simulink model "ee_converter_ultracapacitor"  (R2020a)
settings: Solver=VariableStepAuto  StartTime=0.0  StopTime=15  MaxStep=0.1  RelTol=1e-3  EnableMultiTasking=on
PreLoadFcn:
  | Vref = 12;
StopFcn:
  | ee_addSimlogTimeStamp(bdroot)
libraries: fl_lib x12, nesl_utility x5, ee_lib x3
CloseFcn:
  | try,close(h1_ee_converter_ultracapacitor),end
  | clear h1_ee_converter_ultracapacitor
  | 
  | 
  | clear simlog_ee_converter_ultracapacitor
  | clear logsout_ee_converter_ultracapacitor
  | clear Vref tout
Description:
  | Ultracapacitor With Converter
settings Model: Creator=The MathWorks, Inc.  LastModifiedBy=sateeshk
settings DataIOCC: LimitDataPoints=on  MaxDataPoints=10000  SaveFormat=Array  ReturnWorkspaceOutputs=off  SignalLoggingName=logsout_ee_converter_ultracapacitor
settings OptimizationCC: ExpressionDepthLimit=2147483647  LifeSpan=inf
settings DebuggingCC: UnderspecifiedInitializationDetection=Classic  MergeDetectMultiDrivingBlocksExec=none  SolverPrmCheckMsg=warning  StateNameClashWarn=warning  SFUnexpectedBacktrackingDiag=warning  SFNoUnconditionalDefaultTransitionDiag=warning  SFExecutionAtInitializationDiag=none  ArithmeticOperatorsInVariantConditions=warning
settings HardwareCC: ProdBitPerPointer=32  ProdBitPerSizeT=32  ProdBitPerPtrDiffT=32  ProdLargestAtomicFloat=None  ProdIntDivRoundTo=Undefined  ProdEndianess=Unspecified  ProdWordSize=32  ProdHWDeviceType=32-bit Generic
settings ModelReferenceCC: PropagateSignalLabelsOutOfModel=off
settings SFSimCC: SimUseLocalCustomCode=off  CustomCodeUndefinedFunction=UseInterfaceOnly
settings RTWCC: RTWUseLocalCustomCode=off
settings CodeAppCC: StateflowObjectComments=on
settings GRTTargetCC: TargetLangStandard=C89/C90 (ANSI)
settings ConfigComp: CovMetricSettings=dw  CovHtmlReporting=on  CovSaveCumulativeToWorkspaceVar=on  CovSaveSingleToWorkspaceVar=on  CovExternalEMLEnable=off  CovSFcnEnable=off
settings SimscapeCC: SimscapeLogType=all  SimscapeLogSimulationStatistics=on  SimscapeLogName=simlog_ee_converter_ultracapacitor  SimscapeLogDataHistory=10000

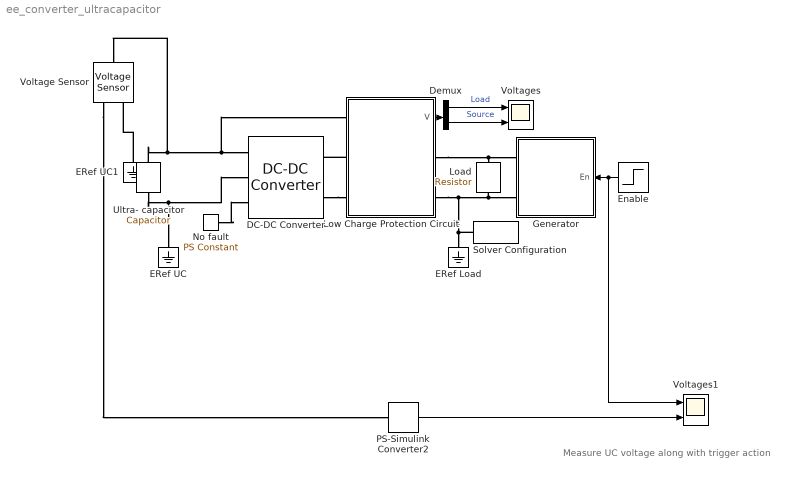
== system ee_converter_ultracapacitor ==
  note: Measure UC voltage along with trigger action
  DC-DC Converter : ee_lib/Semiconductors & Converters/Converters/DC-DC Converter  Vref_option=ee.enum.converters.voltageref.internal  v_ref=Vref V  P_rated=100 W  droop_param=1  droop=0.01 V/A  droop_percent=2  reversible=1  efficiency=95  P_fixed=0.1 W  model_dynamics=0  tau=0.02 s  v_ini=10 V  G_diode=1e-8 1/Ohm  i1_max=100 A  fault_condition=1  fault_threshold=0.5  thermal_mass=100 J/K  initial_temperature=298.15 K
      settings: SourceProductBaseCode=PS  InternalSimscapePortConfiguration="{\"Bottom\":[],\"Left\":[{\"id\":\"p1\",\"label\":\"1+\",\"type\":\"foundation.electrical.electrical\"},{\"id\":\"n1\",\"label\":\"1-\",\"type\":\"foundation.electrical.electrical\"},{\"id\":\"F\",\"label\":\"F\",\"type\":\"input\"}],\"Right\":[{\"id\":\"p2\",\"label\":\"2+\",\"type\":\"foundation.electrical.electrical\"},{\"id\":\"n2\",\"label\":\"2-\",\"type\":\"foundation.electrical.electrical\"}],\"Top\":[]}"
  Demux : Demux  Outputs=2
  ERef Load : fl_lib/Electrical/Electrical Elements/Electrical Reference
      settings: SourceProductBaseCode=MT,SS
  ERef UC : fl_lib/Electrical/Electrical Elements/Electrical Reference
      settings: SourceProductBaseCode=MT,SS
  ERef UC1 : fl_lib/Electrical/Electrical Elements/Electrical Reference
      settings: SourceProductBaseCode=MT,SS
  Enable : Step  Time=5  After=15  SampleTime=0
      settings: AttributesFormatString=On: %<Time> sec
  Generator : Subsystem
  Load : fl_lib/Electrical/Electrical Elements/Resistor  R=2 Ohm  i_specify=off  i_priority=High  i=0 A  i_nominal_specify=off  i_nominal_unit=A  i_nominal_value=1  v_specify=off  v_priority=High  v=0 V  v_nominal_specify=off  v_nominal_unit=V  v_nominal_value=1
      settings: SourceProductBaseCode=MT,SS
  Low Charge Protection Circuit : Subsystem  Tag=PublishSubsystem
  No fault : fl_lib/Physical Signals/Sources/PS Constant  constant=0
      settings: SourceProductBaseCode=MT,SS
  PS-Simulink Converter2 : nesl_utility/PS-Simulink Converter  PhysicalDomain=network_engine_domain  SubClassName=ps_output  LeftPortType=input  RightPortType=output  PseudoPeriodic=off  Frequencies=[]  Unit=1  AffineConversion=off
      settings: SourceProductBaseCode=MT,SS
  Solver Configuration : nesl_utility/Solver Configuration  PhysicalDomain=network_engine_domain  SubClassName=solver  LeftPortType=input  RightPortType=generic  Tones=[]  Harmonics=[]  SimulateNoise=off  Profile=off  UseLocalSampling=off  EnableSwitchedLinearOptims=on  FrequencyDomain=off  UseCCode=off  RelTol=0.001  AbsTol=1e-06  MinStep=1e-09  ToWorkspace=off  RevertToSquareIcSolve=off  NumHomotopyIterations=100  PhasorMode=off  PhasorModeNumHarmonics=1  DoDC=off  ResidualTolerance=1e-9  UseLocalSolver=off  LocalSolverChoice=NE_BACKWARD_EULER_ADVANCER  LocalSolverSampleTime=0.01  DoFixedCost=off  MaxNonlinIter=3  MaxModeIter=2  LinearAlgebra=auto  EquationFormulation=NE_TIME_EF  DelaysMemoryBudget=1024  AutomaticFiltering=on  FilteringTimeConstant=0.001  PartitionStorageMethod=AS_NEEDED  PartitionMemoryBudget=1024  PartitionMethod=FAST
      settings: SourceProductBaseCode=MT,SS
  Ultra- capacitor : fl_lib/Electrical/Electrical Elements/Capacitor  c=10 F  r=0 Ohm  g=0 1/Ohm  i_specify=off  i_priority=High  i=0 A  i_nominal_specify=off  i_nominal_unit=A  i_nominal_value=1  v_specify=off  v_priority=High  v=0 V  v_nominal_specify=off  v_nominal_unit=V  v_nominal_value=1  vc_specify=on  vc_priority=High  vc=10 V  vc_nominal_specify=off  vc_nominal_unit=V  vc_nominal_value=1
      settings: SourceProductBaseCode=MT,SS
  Voltage Sensor : fl_lib/Electrical/Electrical Sensors/Voltage Sensor
  Voltages : Scope  NumInputPorts=2
  Voltages1 : Scope  NumInputPorts=2
  wires:
  Enable/1 -> Voltages1/1, Generator/1(En)
  Low Charge Protection Circuit/1(V) -> Demux/1
  Demux/1 -> Voltages/1  "Load"
  Demux/2 -> Voltages/2  "Source"
  PS-Simulink Converter2/1 -> Voltages1/2
  connections:
  Ultra- capacitor/RConn1 -- DC-DC Converter/LConn2 -- ERef UC/LConn1
  Ultra- capacitor/LConn1 -- Low Charge Protection Circuit/LConn1 -- DC-DC Converter/LConn1 -- Voltage Sensor/LConn1
  Low Charge Protection Circuit/LConn2 -- DC-DC Converter/RConn1
  Low Charge Protection Circuit/RConn2 -- Solver Configuration/RConn1 -- ERef Load/LConn1 -- Generator/RConn2 -- Load/RConn1
  DC-DC Converter/RConn2 -- Low Charge Protection Circuit/LConn3
  Low Charge Protection Circuit/RConn1 -- Load/LConn1 -- Generator/RConn1
  No fault/RConn1 -- DC-DC Converter/LConn3
  ERef UC1/LConn1 -- Voltage Sensor/RConn2
  Voltage Sensor/RConn1 -- PS-Simulink Converter2/LConn1

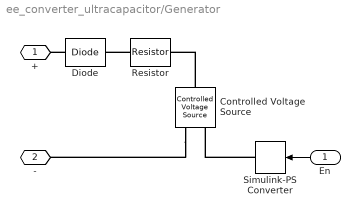
== system ee_converter_ultracapacitor/Generator ==
  En : Inport
  Controlled Voltage Source : fl_lib/Electrical/Electrical Sources/Controlled Voltage Source
      settings: SourceProductBaseCode=MT,SS
  Diode : fl_lib/Electrical/Electrical Elements/Diode  Vf=0.6 V  Ron=0.01 Ohm  Goff=1e-8 1/Ohm  i_specify=off  i_priority=High  i=0 A  i_nominal_specify=off  i_nominal_unit=A  i_nominal_value=1  v_specify=off  v_priority=High  v=0 V  v_nominal_specify=off  v_nominal_unit=V  v_nominal_value=1
      settings: SourceProductBaseCode=MT,SS
  Resistor : fl_lib/Electrical/Electrical Elements/Resistor  R=0.1 Ohm  i_specify=off  i_priority=High  i=0 A  i_nominal_specify=off  i_nominal_unit=A  i_nominal_value=1  v_specify=off  v_priority=High  v=0 V  v_nominal_specify=off  v_nominal_unit=V  v_nominal_value=1
      settings: SourceProductBaseCode=MT,SS
  Simulink-PS Converter : nesl_utility/Simulink-PS Converter  PhysicalDomain=network_engine_domain  SubClassName=ps_input  LeftPortType=input  RightPortType=output  PseudoPeriodic=off  Frequencies=[]  NoiseDistribution=none  NoiseParameters=[]  Unit=1  AffineConversion=off  FilteringAndDerivatives=zero  SimscapeFilterOrder=1  InputFilterTimeConstant=.001  UdotUserProvided=[]
      settings: SourceProductBaseCode=MT,SS
  + : PMIOPort  Side=Right
  - : PMIOPort  Port=2  Side=Right
  wires:
  En/1 -> Simulink-PS Converter/1
  connections:
  Controlled Voltage Source/RConn2 -- -/RConn1
  Simulink-PS Converter/RConn1 -- Controlled Voltage Source/RConn1
  Controlled Voltage Source/LConn1 -- Resistor/LConn1
  Diode/RConn1 -- +/RConn1
  Resistor/RConn1 -- Diode/LConn1

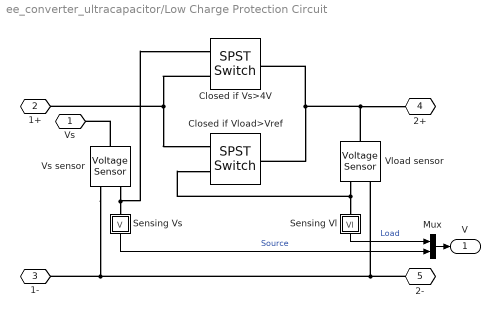
== system ee_converter_ultracapacitor/Low Charge Protection Circuit ==
  Closed if Vload>Vref : ee_lib/Switches & Breakers/SPST Switch  R_closed=0.01 Ohm  G_open=1e-6 S  Threshold=Vref V  Width=0.1 V  model_dynamics=0  t_on=0.001 s  t_off=0.001 s  initial_vT=0 V
      settings: SourceProductBaseCode=PS  InternalSimscapePortConfiguration="{\"Bottom\":[],\"Left\":[{\"id\":\"vT\",\"label\":\"vT\",\"type\":\"input\"},{\"id\":\"p\",\"label\":\"\",\"type\":\"foundation.electrical.electrical\"}],\"Right\":[{\"id\":\"n\",\"label\":\"\",\"type\":\"foundation.electrical.electrical\"}],\"Top\":[]}"
  Closed if Vs>4V : ee_lib/Switches & Breakers/SPST Switch  R_closed=0.01 Ohm  G_open=1e-6 S  Threshold=4 V  Width=0.1 V  model_dynamics=0  t_on=0.001 s  t_off=0.001 s  initial_vT=0 V
      settings: SourceProductBaseCode=PS  InternalSimscapePortConfiguration="{\"Bottom\":[],\"Left\":[{\"id\":\"vT\",\"label\":\"vT\",\"type\":\"input\"},{\"id\":\"p\",\"label\":\"\",\"type\":\"foundation.electrical.electrical\"}],\"Right\":[{\"id\":\"n\",\"label\":\"\",\"type\":\"foundation.electrical.electrical\"}],\"Top\":[]}"
  Mux : Mux  Inputs=2
  Sensing Vl : Subsystem
      mask Display: disp('Vl')
  Sensing Vs : Subsystem
      mask Display: disp('Vs')
  Vload sensor : fl_lib/Electrical/Electrical Sensors/Voltage Sensor
      settings: SourceProductBaseCode=MT,SS
  Vs sensor : fl_lib/Electrical/Electrical Sensors/Voltage Sensor
      settings: SourceProductBaseCode=MT,SS
  Vs : PMIOPort  Side=Left
  1+ : PMIOPort  Port=2  Side=Left
  1- : PMIOPort  Port=3  Side=Left
  2+ : PMIOPort  Port=4  Side=Right
  2- : PMIOPort  Port=5  Side=Right
  V : Outport  VectorParamsAs1DForOutWhenUnconnected=off
  wires:
  Sensing Vl/1(Vl) -> Mux/1  "Load"
  Mux/1 -> V/1
  Sensing Vs/1(V) -> Mux/2  "Source"
  connections:
  Vload sensor/LConn1 -- 2+/RConn1 -- Closed if Vload>Vref/RConn1 -- Closed if Vs>4V/RConn1
  2-/RConn1 -- Vload sensor/RConn2 -- Vs sensor/RConn2 -- 1-/RConn1
  Closed if Vs>4V/LConn2 -- Closed if Vload>Vref/LConn2 -- 1+/RConn1
  Vs sensor/LConn1 -- Vs/RConn1
  Vs sensor/RConn1 -- Closed if Vs>4V/LConn1 -- Sensing Vs/LConn1
  Vload sensor/RConn1 -- Closed if Vload>Vref/LConn1 -- Sensing Vl/LConn1

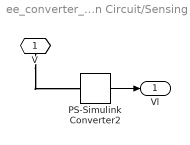
== system ee_converter_ultracapacitor/Low Charge Protection Circuit/Sensing Vl ==
  PS-Simulink Converter2 : nesl_utility/PS-Simulink Converter  PhysicalDomain=network_engine_domain  SubClassName=ps_output  LeftPortType=input  RightPortType=output  PseudoPeriodic=off  Frequencies=[]  Unit=1  AffineConversion=off
      settings: SourceProductBaseCode=MT,SS
  V : PMIOPort  Side=Left
  Vl : Outport  VectorParamsAs1DForOutWhenUnconnected=off
  wires:
  PS-Simulink Converter2/1 -> Vl/1
  connections:
  V/RConn1 -- PS-Simulink Converter2/LConn1

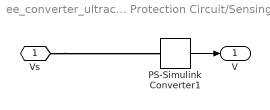
== system ee_converter_ultracapacitor/Low Charge Protection Circuit/Sensing Vs ==
  PS-Simulink Converter1 : nesl_utility/PS-Simulink Converter  PhysicalDomain=network_engine_domain  SubClassName=ps_output  LeftPortType=input  RightPortType=output  PseudoPeriodic=off  Frequencies=[]  Unit=1  AffineConversion=off
      settings: SourceProductBaseCode=MT,SS
  Vs : PMIOPort  Side=Left
  V : Outport  VectorParamsAs1DForOutWhenUnconnected=off
  wires:
  PS-Simulink Converter1/1 -> V/1
  connections:
  Vs/RConn1 -- PS-Simulink Converter1/LConn1
